simulink model "Calcul_Transfert_Mono"  (R2020b)
settings: Solver=VariableStepAuto  StartTime=0.0  StopTime=10.0  RelTol=1e-3
undefined symbols (not defined in the file or in its folder): A, A_K1, B, B_K1, C, C_K1, D, D_K1
settings Model: Creator=Sandou  LastModifiedBy=Sandou

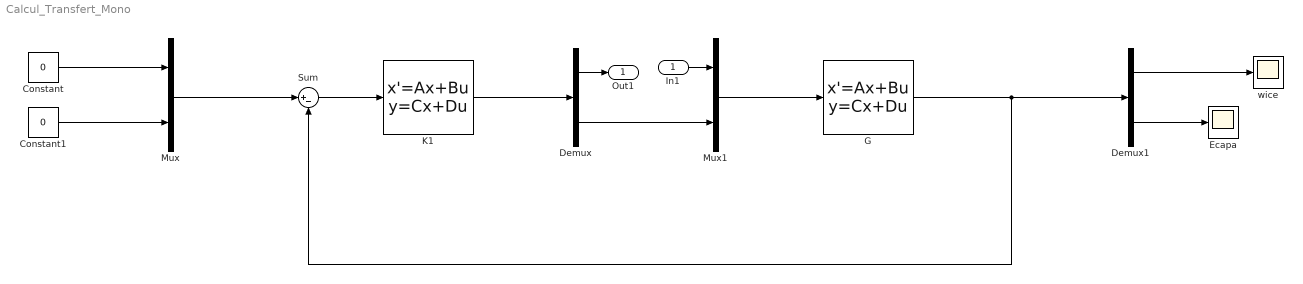
== system Calcul_Transfert_Mono ==
  In1 : Inport
  Constant : Constant  Value=0
  Constant1 : Constant  Value=0
  Demux : Demux  Outputs=2
  Demux1 : Demux  Outputs=2
  Ecapa : Scope
  G : StateSpace  A=A  B=B  C=C  D=D  InitialCondition=0
  K1 : StateSpace  A=A_K1  B=B_K1  C=C_K1  D=D_K1  InitialCondition=0
  Mux : Mux  Inputs=2
  Mux1 : Mux  Inputs=2
  Sum : Sum  Inputs=|+-
  wice : Scope
  Out1 : Outport
  wires:
  K1/1 -> Demux/1
  Sum/1 -> K1/1
  G/1 -> Demux1/1, Sum/2
  Mux/1 -> Sum/1
  Constant/1 -> Mux/1
  Constant1/1 -> Mux/2
  Demux1/1 -> wice/1
  Demux1/2 -> Ecapa/1
  Mux1/1 -> G/1
  Demux/2 -> Mux1/2
  Demux/1 -> Out1/1
  In1/1 -> Mux1/1
